simulink model "TBRe19_ECU_SequentialTests"  (R2017b)
settings: Solver=FixedStepDiscrete  StartTime=0.0  StopTime=inf  FixedStep=0.0001  RelTol=1e-3
PostLoadFcn:
  | model_init();
libraries: simulink x28
(part 2 of 22)

== system TBRe19_ECU_SequentialTests/DiagCAN3 ==
  note: ECU_Diag_ToCAN
  PostPL_Bus : Inport
  Bus Selector : BusSelector  OutputSignals=VFL_Data.DAL_Data.HAL_Data.HAL_Hardwired.Throttle1_Voltage,VFL_Data.DAL_Data.HAL_Data.HAL_Hardwired.Throttle2_Voltage,VFL_Data.DAL_Data.HAL_Data.HAL_Hardwired.Brake1_Pressure,VFL_Data.DAL_Data.HAL_Data.HAL_Hardwired.Brake2_Pressure
  Bus Selector1 : BusSelector  OutputSignals=VFL_Data.DAL_Data.Pedal_Box_Data.Brake1_Per,VFL_Data.DAL_Data.Pedal_Box_Data.Brake2_Per,VFL_Data.DAL_Data.Pedal_Box_Data.Brake_Percentage,VFL_Data.DAL_Data.Pedal_Box_Data.Throttle1_Per,VFL_Data.DAL_Data.Pedal_Box_Data.Throttle2_Per,VFL_Data.DAL_Data.Pedal_Box_Data.Throttle_Percentage
  Bus Selector2 : BusSelector  OutputSignals=VFL_Data.DAL_Data.HAL_Data.HAL_Hardwired.btnRTD_Input,VFL_Data.DAL_Data.HAL_Data.HAL_Hardwired.btnX_Input,VFL_Data.DAL_Data.HAL_Data.HAL_Hardwired.btnY_Input,VFL_Data.DAL_Data.HAL_Data.HAL_Hardwired.btnZ_Input,VFL_Data.DAL_Data.HAL_Data.HAL_Hardwired.Fan_Freq
  Bus Selector3 : BusSelector  OutputSignals=VFL_Data.DAL_Data.Pedal_Box_Data.Throttle_Bool,VFL_Data.DAL_Data.Pedal_Box_Data.Brake_Bool
  Bus Selector4 : BusSelector  OutputSignals=VFL_Data.DAL_Data.HAL_Data.HAL_Hardwired.AIRLow,VFL_Data.DAL_Data.HAL_Data.HAL_Hardwired.AIRHigh,VFL_Data.DAL_Data.Pedal_Box_Data.BPPS_Implausibility,VFL_Data.DAL_Data.Pedal_Box_Data.Pedal_Sensor_Fail,VFL_Data.DAL_Data.Pedal_Box_Data.APPS_Implausibility,VFL_Data.DAL_Data.Pedal_Box_Data.APPS_BP_Implausibility
  CanTx2 : S-Function  FunctionName=NsiCan_Tx_Ext  Parameters=data_can,channel,msg_name,ident,ident_type,dlc,signals,is_physical,is_canfd,is_crc  SFunctionDeploymentMode=off  EnableBusSupport=off  mask(MUXlink Can Tx){data_can=1;HIGH_SPEED;500Kbps;No;C:\Users\TBRe-admin\Documents\Database\TBRe19_DBC_190620.dbc;0;;;0;HIGH_SPEED;500Kbps;120 Ohm;C:\Users\TBRe-admin\Documents\Database\TBRe19_DBC_190517.dbc;0;;;0;HIGH_SPEED;1000Kbps;120 Ohm;D:\TOOLS\MUXLINK\R2011b\MUXlink\misc\BASE_CAN_MUXLAB4.dbc;0;;;0;HIGH_SPEED;500Kbps;120 Ohm;D:\TOOLS\MUXLINK\R2011b\MUXlink\misc\j1939_adapt.dbc;0;;;0;HIGH_SPEED;1000Kbps;No;D:\TOOLS\MUXLINK\R2011b\MUXlink\misc\BASE_CAN_MUXLAB4.dbc;0;;, channel=1, msg_name=VCU_Diagnostics, ident=0x700, ident_type=STD, dlc=4, signals=Shutdown_ECU;1;22;-1;1.000000;0.000000;_;Low_AIR_Status;1;20;-1;1.000000;0.000000;_;High_AIR_Status;1;21;1;1.000000;0.000000;_;BPPS_Implausibility;1;16;-1;1.000000;0.000000;_;Pedal_Sensor_Fail;1;24;8;1.000000;0.000000;_;APPS_Implausibility;1;17;1;1.000000;0.000000;_;APPS_BP_Implausibility;1;18;1;1.000000;0.000000;_;Shutdown_CarShutdown;1;23;1;1.000000;0.000000;_;LV_Battery_Warning;1;19;1;1.000000;0.000000;_;GearingRatio;1;8;8;0.100000;0.000000;_;Wheel_Size;1;0;8;0.100000;0.000000;m;Boost_on;1;34;-1;1.000000;0.000000;_;TC_on;1;33;-1;1.000000;0.000000;_;RegenBool;1;32;-1;1.000000;0.000000;_, is_physical=0, is_canfd=0, is_crc=0}
      mask prompts: data_can "data can"; msg_name "msg name"
      mask help: Transmit a frame on a CAN Channel.
      mask init:
      | NsiCan_Tx_Ext_InitializationFcn();
      settings: OpenFcn=NsiCan_Tx_Ext_OpenFcn();
      mask Help:
      | eval('block=get_param(gcb, ''RTWdata'');')
      | web([docroot '\toolbox\MUXlink\html\blocks/' block.MUXlink_BlockType '.html'])
      mask Callback data_can: NsiCan_Tx_Ext_ApplyFcn(1);
      mask Callback channel: NsiCan_Tx_Ext_ApplyFcn(2);
      mask Callback msg_name: NsiCan_Tx_Ext_ApplyFcn(3);
      mask Callback ident: NsiCan_Tx_Ext_ApplyFcn(4);
      mask Callback ident_type: NsiCan_Tx_Ext_ApplyFcn(5);
      mask Callback dlc: NsiCan_Tx_Ext_ApplyFcn(6);
      mask Callback signals: NsiCan_Tx_Ext_ApplyFcn(7);
      mask Callback is_physical: NsiCan_Tx_Ext_ApplyFcn(7);
      mask Callback is_canfd: NsiCan_Tx_Ext_ApplyFcn(7);
      mask Callback is_crc: NsiCan_Tx_Ext_ApplyFcn(7);
      mask Display: image(imread('nsi.bmp'));text(0.5, 0.3, 'TX_VCU_Diagnostics_CAN1', 'horizontalAlignment', 'center', 'verticalAlignment', 'base');plot([0.05 0.05 0.05 0.05 0.05 0.05 0.05 0.05 0.05 0.05]); port_label('input',1, 'Shutdown_ECU'); port_label('input',2, 'Low_AIR_Status'); port_label('input',3, 'High_AIR_Status'); port_label('input',4, 'BPPS_Implausibility'); port_label('input',5, 'Pedal_Sensor_Fail'); port_label('input',6, 'APPS_Implausibility'); port_label('input',7, 'APPS_BP_Implausibility'); port_label('input',8, 'Shutdown_CarShutdown'); port_label('input',9, 'LV_Battery_Warning'); port_label('input',10, 'GearingRatio'); port_label('input',11, 'Wheel_Size'); port_label('input',12, 'Boost_on'); port_label('input',13, 'TC_on'); port_label('input',14, 'RegenBool');
  CanTx6 : S-Function  FunctionName=NsiCan_Tx_Ext  Parameters=data_can,channel,msg_name,ident,ident_type,dlc,signals,is_physical,is_canfd,is_crc  SFunctionDeploymentMode=off  EnableBusSupport=off  mask(MUXlink Can Tx){data_can=1;HIGH_SPEED;500Kbps;No;C:\Users\TBRe-admin\Documents\Database\TBRe19_DBC_190621.dbc;0;;;0;HIGH_SPEED;500Kbps;120 Ohm;C:\Users\TBRe-admin\Documents\Database\TBRe19_DBC_190517.dbc;0;;;0;HIGH_SPEED;1000Kbps;120 Ohm;D:\TOOLS\MUXLINK\R2011b\MUXlink\misc\BASE_CAN_MUXLAB4.dbc;0;;;0;HIGH_SPEED;500Kbps;120 Ohm;D:\TOOLS\MUXLINK\R2011b\MUXlink\misc\j1939_adapt.dbc;0;;;0;HIGH_SPEED;1000Kbps;No;D:\TOOLS\MUXLINK\R2011b\MUXlink\misc\BASE_CAN_MUXLAB4.dbc;0;;, channel=1, msg_name=VCU_Pedal_Percentages, ident=0x702, ident_type=STD, dlc=7, signals=Brake1_Percentage;1;24;8;1.000000;0.000000;%;Brake2_Percentage;1;32;8;1.000000;0.000000;%;Brake_Percentage;1;48;8;1.000000;0.000000;%;BrakePot_Percentage;1;40;8;1.000000;0.000000;%;Throttle1_Percent;1;0;8;1.000000;0.000000;%;Throttle2_Percentage;1;8;8;1.000000;0.000000;%;Throttle_Percentage;1;16;8;1.000000;0.000000;%, is_physical=0, is_canfd=0, is_crc=0}
      mask prompts: data_can "data can"; msg_name "msg name"
      mask help: Transmit a frame on a CAN Channel.
      mask init:
      | NsiCan_Tx_Ext_InitializationFcn();
      settings: OpenFcn=NsiCan_Tx_Ext_OpenFcn();
      mask Help:
      | eval('block=get_param(gcb, ''RTWdata'');')
      | web([docroot '\toolbox\MUXlink\html\blocks/' block.MUXlink_BlockType '.html'])
      mask Callback data_can: NsiCan_Tx_Ext_ApplyFcn(1);
      mask Callback channel: NsiCan_Tx_Ext_ApplyFcn(2);
      mask Callback msg_name: NsiCan_Tx_Ext_ApplyFcn(3);
      mask Callback ident: NsiCan_Tx_Ext_ApplyFcn(4);
      mask Callback ident_type: NsiCan_Tx_Ext_ApplyFcn(5);
      mask Callback dlc: NsiCan_Tx_Ext_ApplyFcn(6);
      mask Callback signals: NsiCan_Tx_Ext_ApplyFcn(7);
      mask Callback is_physical: NsiCan_Tx_Ext_ApplyFcn(7);
      mask Callback is_canfd: NsiCan_Tx_Ext_ApplyFcn(7);
      mask Callback is_crc: NsiCan_Tx_Ext_ApplyFcn(7);
      mask Display: image(imread('nsi.bmp'));text(0.5, 0.1, 'TX_VCU_Pedal_Percentages_CAN1', 'horizontalAlignment', 'center', 'verticalAlignment', 'base');plot([0.05 0.05 0.05 0.05 0.05 0.05 0.05 0.05 0.05 0.05]); port_label('input',1, 'Brake1_Percentage'); port_label('input',2, 'Brake2_Percentage'); port_label('input',3, 'Brake_Percentage'); port_label('input',4, 'BrakePot_Percentage'); port_label('input',5, 'Throttle1_Percent'); port_label('input',6, 'Throttle2_Percentage'); port_label('input',7, 'Throttle_Percentage');
  CanTx7 : S-Function  FunctionName=NsiCan_Tx_Ext  Parameters=data_can,channel,msg_name,ident,ident_type,dlc,signals,is_physical,is_canfd,is_crc  SFunctionDeploymentMode=off  EnableBusSupport=off  mask(MUXlink Can Tx){data_can=1;HIGH_SPEED;500Kbps;No;C:\Users\TBRe-admin\Documents\Database\TBRe19_DBC_190621.dbc;0;;;0;HIGH_SPEED;500Kbps;120 Ohm;C:\Users\TBRe-admin\Documents\Database\TBRe19_DBC_190517.dbc;0;;;0;HIGH_SPEED;1000Kbps;120 Ohm;D:\TOOLS\MUXLINK\R2011b\MUXlink\misc\BASE_CAN_MUXLAB4.dbc;0;;;0;HIGH_SPEED;500Kbps;120 Ohm;D:\TOOLS\MUXLINK\R2011b\MUXlink\misc\j1939_adapt.dbc;0;;;0;HIGH_SPEED;1000Kbps;No;D:\TOOLS\MUXLINK\R2011b\MUXlink\misc\BASE_CAN_MUXLAB4.dbc;0;;, channel=1, msg_name=VCU_HW_IO, ident=0x701, ident_type=STD, dlc=4, signals=Console_RTD;1;0;1;1.000000;0.000000;Bool;Console_X;1;3;1;1.000000;0.000000;Bool;Consle_Y;1;2;-1;1.000000;0.000000;Bool;Console_Z;1;1;-1;1.000000;0.000000;_;Coolant_Pump_Fan;1;5;1;1.000000;0.000000;_;Coolant_AccyFan;1;6;-1;1.000000;0.000000;_;Buzzer;1;7;1;1.000000;0.000000;_;LV_Battery_Voltage;1;16;16;1.000000;0.000000;mV;LV_Battery_SOC;1;8;8;1.000000;0.000000;_;AccyFanFreq;1;32;8;1.000000;0.000000;Hz, is_physical=0, is_canfd=0, is_crc=0}
      mask prompts: data_can "data can"; msg_name "msg name"
      mask help: Transmit a frame on a CAN Channel.
      mask init:
      | NsiCan_Tx_Ext_InitializationFcn();
      settings: OpenFcn=NsiCan_Tx_Ext_OpenFcn();
      mask Help:
      | eval('block=get_param(gcb, ''RTWdata'');')
      | web([docroot '\toolbox\MUXlink\html\blocks/' block.MUXlink_BlockType '.html'])
      mask Callback data_can: NsiCan_Tx_Ext_ApplyFcn(1);
      mask Callback channel: NsiCan_Tx_Ext_ApplyFcn(2);
      mask Callback msg_name: NsiCan_Tx_Ext_ApplyFcn(3);
      mask Callback ident: NsiCan_Tx_Ext_ApplyFcn(4);
      mask Callback ident_type: NsiCan_Tx_Ext_ApplyFcn(5);
      mask Callback dlc: NsiCan_Tx_Ext_ApplyFcn(6);
      mask Callback signals: NsiCan_Tx_Ext_ApplyFcn(7);
      mask Callback is_physical: NsiCan_Tx_Ext_ApplyFcn(7);
      mask Callback is_canfd: NsiCan_Tx_Ext_ApplyFcn(7);
      mask Callback is_crc: NsiCan_Tx_Ext_ApplyFcn(7);
      mask Display: image(imread('nsi.bmp'));text(0.5, 0.3, 'TX_VCU_HW_IO_CAN1', 'horizontalAlignment', 'center', 'verticalAlignment', 'base');plot([0.05 0.05 0.05 0.05 0.05 0.05 0.05 0.05 0.05 0.05]); port_label('input',1, 'Console_RTD'); port_label('input',2, 'Console_X'); port_label('input',3, 'Consle_Y'); port_label('input',4, 'Console_Z'); port_label('input',5, 'Coolant_Pump_Fan'); port_label('input',6, 'Coolant_AccyFan'); port_label('input',7, 'Buzzer'); port_label('input',8, 'LV_Battery_Voltage'); port_label('input',9, 'LV_Battery_SOC'); port_label('input',10, 'AccyFanFreq');
  CanTx8 : S-Function  FunctionName=NsiCan_Tx_Ext  Parameters=data_can,channel,msg_name,ident,ident_type,dlc,signals,is_physical,is_canfd,is_crc  SFunctionDeploymentMode=off  EnableBusSupport=off  mask(MUXlink Can Tx){data_can=1;HIGH_SPEED;500Kbps;No;C:\Users\TBRe-admin\Documents\Database\TBRe19_DBC_190620.dbc;0;;;0;HIGH_SPEED;500Kbps;120 Ohm;C:\Users\TBRe-admin\Documents\Database\TBRe19_DBC_190517.dbc;0;;;0;HIGH_SPEED;1000Kbps;120 Ohm;D:\TOOLS\MUXLINK\R2011b\MUXlink\misc\BASE_CAN_MUXLAB4.dbc;0;;;0;HIGH_SPEED;500Kbps;120 Ohm;D:\TOOLS\MUXLINK\R2011b\MUXlink\misc\j1939_adapt.dbc;0;;;0;HIGH_SPEED;1000Kbps;No;D:\TOOLS\MUXLINK\R2011b\MUXlink\misc\BASE_CAN_MUXLAB4.dbc;0;;, channel=1, msg_name=VCU_Vehicle_Functionality, ident=0x704, ident_type=STD, dlc=4, signals=Tractive_System_Startup;1;24;1;1.000000;0.000000;_;Throttle_Bool;1;25;1;1.000000;0.000000;_;MCU_NMT_Mode;1;16;8;1.000000;0.000000;_;Control_Word;1;0;8;1.000000;0.000000;_;Vehicle_Operation;1;8;8;1.000000;0.000000;_;Brake_Bool;1;26;1;1.000000;0.000000;_, is_physical=0, is_canfd=0, is_crc=0}
      mask prompts: data_can "data can"; msg_name "msg name"
      mask help: Transmit a frame on a CAN Channel.
      mask init:
      | NsiCan_Tx_Ext_InitializationFcn();
      settings: OpenFcn=NsiCan_Tx_Ext_OpenFcn();
      mask Help:
      | eval('block=get_param(gcb, ''RTWdata'');')
      | web([docroot '\toolbox\MUXlink\html\blocks/' block.MUXlink_BlockType '.html'])
      mask Callback data_can: NsiCan_Tx_Ext_ApplyFcn(1);
      mask Callback channel: NsiCan_Tx_Ext_ApplyFcn(2);
      mask Callback msg_name: NsiCan_Tx_Ext_ApplyFcn(3);
      mask Callback ident: NsiCan_Tx_Ext_ApplyFcn(4);
      mask Callback ident_type: NsiCan_Tx_Ext_ApplyFcn(5);
      mask Callback dlc: NsiCan_Tx_Ext_ApplyFcn(6);
      mask Callback signals: NsiCan_Tx_Ext_ApplyFcn(7);
      mask Callback is_physical: NsiCan_Tx_Ext_ApplyFcn(7);
      mask Callback is_canfd: NsiCan_Tx_Ext_ApplyFcn(7);
      mask Callback is_crc: NsiCan_Tx_Ext_ApplyFcn(7);
      mask Display: image(imread('nsi.bmp'));text(0.5, 0.3, 'TX_VCU_Vehicle_Functionality_CAN1', 'horizontalAlignment', 'center', 'verticalAlignment', 'base');plot([0.05 0.05 0.05 0.05 0.05 0.05 0.05 0.05 0.05 0.05]); port_label('input',1, 'Tractive_System_Startup'); port_label('input',2, 'Throttle_Bool'); port_label('input',3, 'MCU_NMT_Mode'); port_label('input',4, 'Control_Word'); port_label('input',5, 'Vehicle_Operation'); port_label('input',6, 'Brake_Bool');
  CanTx9 : S-Function  FunctionName=NsiCan_Tx_Ext  Parameters=data_can,channel,msg_name,ident,ident_type,dlc,signals,is_physical,is_canfd,is_crc  SFunctionDeploymentMode=off  EnableBusSupport=off  mask(MUXlink Can Tx){data_can=1;HIGH_SPEED;500Kbps;No;C:\Users\TBRe-admin\Documents\Database\TBRe19_DBC_190621.dbc;0;;;0;HIGH_SPEED;500Kbps;120 Ohm;C:\Users\TBRe-admin\Documents\Database\TBRe19_DBC_190517.dbc;0;;;0;HIGH_SPEED;1000Kbps;120 Ohm;D:\TOOLS\MUXLINK\R2011b\MUXlink\misc\BASE_CAN_MUXLAB4.dbc;0;;;0;HIGH_SPEED;500Kbps;120 Ohm;D:\TOOLS\MUXLINK\R2011b\MUXlink\misc\j1939_adapt.dbc;0;;;0;HIGH_SPEED;1000Kbps;No;D:\TOOLS\MUXLINK\R2011b\MUXlink\misc\BASE_CAN_MUXLAB4.dbc;0;;, channel=1, msg_name=VCU_Pedal_Voltages, ident=0x703, ident_type=STD, dlc=8, signals=Throttle1_Voltage;1;0;16;1.000000;0.000000;mV;Throttle2_Voltage;1;32;16;1.000000;0.000000;mV;Brake1_Voltage;1;16;16;1.000000;0.000000;mV;Brake2_Voltage;1;48;16;1.000000;0.000000;mV, is_physical=0, is_canfd=0, is_crc=0}
      mask prompts: data_can "data can"; msg_name "msg name"
      mask help: Transmit a frame on a CAN Channel.
      mask init:
      | NsiCan_Tx_Ext_InitializationFcn();
      settings: OpenFcn=NsiCan_Tx_Ext_OpenFcn();
      mask Help:
      | eval('block=get_param(gcb, ''RTWdata'');')
      | web([docroot '\toolbox\MUXlink\html\blocks/' block.MUXlink_BlockType '.html'])
      mask Callback data_can: NsiCan_Tx_Ext_ApplyFcn(1);
      mask Callback channel: NsiCan_Tx_Ext_ApplyFcn(2);
      mask Callback msg_name: NsiCan_Tx_Ext_ApplyFcn(3);
      mask Callback ident: NsiCan_Tx_Ext_ApplyFcn(4);
      mask Callback ident_type: NsiCan_Tx_Ext_ApplyFcn(5);
      mask Callback dlc: NsiCan_Tx_Ext_ApplyFcn(6);
      mask Callback signals: NsiCan_Tx_Ext_ApplyFcn(7);
      mask Callback is_physical: NsiCan_Tx_Ext_ApplyFcn(7);
      mask Callback is_canfd: NsiCan_Tx_Ext_ApplyFcn(7);
      mask Callback is_crc: NsiCan_Tx_Ext_ApplyFcn(7);
      mask Display: image(imread('nsi.bmp'));text(0.5, 0.3, 'TX_VCU_Pedal_Voltages_CAN1', 'horizontalAlignment', 'center', 'verticalAlignment', 'base');plot([0.05 0.05 0.05 0.05 0.05 0.05 0.05 0.05 0.05 0.05]); port_label('input',1, 'Throttle1_Voltage'); port_label('input',2, 'Throttle2_Voltage'); port_label('input',3, 'Brake1_Voltage'); port_label('input',4, 'Brake2_Voltage');
  Data Type Conversion{2..11,14,17,21..22,26..30} (19 alike) : DataTypeConversion
  Init : Subsystem  mask(System Initialize){}
      mask help: Add code to a systems Initialize function
      settings: CopyFcn=cccopyfcn(gcb)  OpenFcn=ccopenfcn('System Initialize Function')
      mask Help: This block contains text fields to insert custom user code sections at the declaration, execution and exit sections of the systems initialize function.  By placing this block inside a subsytem, the custom user code will appear in that subsystems function.
      mask Display: disp('I()')
  Task : S-Function  FunctionName=NsiSys_TaskREF  Parameters=task_initialised,task_periodic, task_sampletime,task_name,task_event,task_offset  SFunctionDeploymentMode=off  EnableBusSupport=off  mask(task definition){task_initialised=on, task_periodic=on, task_sampletime=[0.1], task_offset=0.01, task_name=DiagCAN3, task_event=on}
      mask prompts: task_initialised "task initialised"; task_periodic "Is Periodic"; task_sampletime "Task sample time"; task_offset "Task Offset"; task_name "Task name"; task_event "Is event"
      mask help:
      | Permit to provide all parameters associated to a MUXLINK task.
      | Task can be executed periodicaly and/or on event detection.
      | If task is periodic:
      | Task sample time specify the execution period in mS [0.001   6000]
      | Task Offset specify the offset applied to the execution period
      | Task Offset < Task sample time
      mask init:
      | NsiSys_TaskREF_InitializationFcn();
      settings: OpenFcn=NsiSys_Task_OpenFcn();
      mask Callback task_initialised: NsiSys_TaskREF_ApplyFcn(1);
      mask Callback task_periodic: NsiSys_TaskREF_ApplyFcn(2);
      mask Callback task_sampletime: NsiSys_TaskREF_ApplyFcn(3);
      mask Callback task_offset: NsiSys_TaskREF_ApplyFcn(6);
      mask Callback task_name: NsiSys_TaskREF_ApplyFcn(4);
      mask Callback task_event: NsiSys_TaskREF_ApplyFcn(5);
      mask Display: text(0.5, 0.8, 't()', 'horizontalAlignment', 'center', 'verticalAlignment', 'base');text(0.5, 0.2, '/ 100.0ms / 10.0ms /', 'horizontalAlignment', 'center', 'verticalAlignment', 'base');text(0.5, 0.4, 'Event', 'horizontalAlignment', 'center', 'verticalAlignment', 'base');
  UsbRx : S-Function  FunctionName=NsiUsb_Rx  Parameters=signame,sigtype,resolution,offset,unite,value,is_trigger  SFunctionDeploymentMode=off  EnableBusSupport=off  mask(MUXlink Usb Rx){signame=Wheel_Size, sigtype=Unsigned Byte, resolution=1, offset=0, unite=mm, value=450, is_trigger=off}
      mask prompts: signame "Signal name :"; sigtype "Signal type :"; resolution "Resolution :"; offset "Offset :"; unite "Unit :"; value "Default value :"; is_trigger "Is trigger ?"
      mask help: Receive a frame on the USB Channel.
      mask init:
      | NsiUsb_Rx_InitializationFcn();
      settings: OpenFcn=NsiUsb_Rx_OpenFcn();
      mask Help:
      | eval('block=get_param(gcb, ''RTWdata'');')
      | web([docroot '\toolbox\MUXlink\html\blocks/' block.MUXlink_BlockType '.html'])
      mask Callback signame: NsiUsb_Rx_ApplyFcn(1);
      mask TypeOptions sigtype: Boolean | Signed Byte | Unsigned Byte | Signed Word | Unsigned Word | Signed Double Word | Unsigned Double Word | Single Float | Double Float
      mask Callback sigtype: NsiUsb_Rx_ApplyFcn(2);
      mask Callback resolution: NsiUsb_Rx_ApplyFcn(3);
      mask Callback offset: NsiUsb_Rx_ApplyFcn(4);
      mask Callback unite: NsiUsb_Rx_ApplyFcn(5);
      mask Callback value: NsiUsb_Rx_ApplyFcn(6);
      mask Callback is_trigger: NsiUsb_Rx_ApplyFcn(7);
      mask Display: image(imread('nsi.bmp'));text(0.5, 0.2, 'USB Rx', 'horizontalAlignment', 'center', 'verticalAlignment', 'base');plot([0.05 0.05 0.05 0.05 0.05 0.05 0.05 0.05 0.05 0.05]);port_label('output',1, 'Wheel_Size');
  UsbRx1 : S-Function  FunctionName=NsiUsb_Rx  Parameters=signame,sigtype,resolution,offset,unite,value,is_trigger  SFunctionDeploymentMode=off  EnableBusSupport=off  mask(MUXlink Usb Rx){signame=Gearing_Ratio, sigtype=Unsigned Byte, resolution=1, offset=0, unite=ratio, value=3, is_trigger=off}
      mask prompts: signame "Signal name :"; sigtype "Signal type :"; resolution "Resolution :"; offset "Offset :"; unite "Unit :"; value "Default value :"; is_trigger "Is trigger ?"
      mask help: Receive a frame on the USB Channel.
      mask init:
      | NsiUsb_Rx_InitializationFcn();
      settings: OpenFcn=NsiUsb_Rx_OpenFcn();
      mask Help:
      | eval('block=get_param(gcb, ''RTWdata'');')
      | web([docroot '\toolbox\MUXlink\html\blocks/' block.MUXlink_BlockType '.html'])
      mask Callback signame: NsiUsb_Rx_ApplyFcn(1);
      mask TypeOptions sigtype: Boolean | Signed Byte | Unsigned Byte | Signed Word | Unsigned Word | Signed Double Word | Unsigned Double Word | Single Float | Double Float
      mask Callback sigtype: NsiUsb_Rx_ApplyFcn(2);
      mask Callback resolution: NsiUsb_Rx_ApplyFcn(3);
      mask Callback offset: NsiUsb_Rx_ApplyFcn(4);
      mask Callback unite: NsiUsb_Rx_ApplyFcn(5);
      mask Callback value: NsiUsb_Rx_ApplyFcn(6);
      mask Callback is_trigger: NsiUsb_Rx_ApplyFcn(7);
      mask Display: image(imread('nsi.bmp'));text(0.5, 0.2, 'USB Rx', 'horizontalAlignment', 'center', 'verticalAlignment', 'base');plot([0.05 0.05 0.05 0.05 0.05 0.05 0.05 0.05 0.05 0.05]);port_label('output',1, 'Gearing_Ratio');
  wires:
  Data Type Conversion17/1 -> CanTx8/2
  Data Type Conversion14/1 -> CanTx6/1
  Data Type Conversion22/1 -> CanTx7/10
  Data Type Conversion28/1 -> CanTx2/4
  Data Type Conversion26/1 -> CanTx2/3
  Data Type Conversion6/1 -> CanTx9/4
  Data Type Conversion11/1 -> CanTx2/5
  Data Type Conversion3/1 -> CanTx9/3
  Data Type Conversion4/1 -> CanTx9/1
  Bus Selector1/6 -> Data Type Conversion5/1  "<Throttle_Percentage>"
  Data Type Conversion21/1 -> CanTx8/6
  Bus Selector/4 -> Data Type Conversion6/1  "<Brake2_Pressure>"
  UsbRx1/1 -> CanTx2/10
  Bus Selector2/4 -> CanTx7/4  "<btnZ_Input>"
  Bus Selector4/3 -> Data Type Conversion28/1  "<BPPS_Implausibility>"
  Bus Selector4/1 -> Data Type Conversion27/1  "<AIRLow>"
  Data Type Conversion9/1 -> CanTx6/6
  Bus Selector1/1 -> Data Type Conversion14/1  "<Brake1_Per>"
  UsbRx/1 -> CanTx2/11
  Bus Selector4/2 -> Data Type Conversion26/1  "<AIRHigh>"
  Data Type Conversion27/1 -> CanTx2/2
  Data Type Conversion29/1 -> CanTx2/6
  Data Type Conversion5/1 -> CanTx6/7
  Data Type Conversion7/1 -> CanTx6/2
  Data Type Conversion8/1 -> CanTx6/3
  Bus Selector1/3 -> Data Type Conversion8/1  "<Brake_Percentage>"
  Bus Selector4/6 -> Data Type Conversion30/1  "<APPS_BP_Implausibility>"
  Bus Selector/1 -> Data Type Conversion4/1  "<Throttle1_Voltage>"
  Bus Selector4/5 -> Data Type Conversion29/1  "<APPS_Implausibility>"
  Bus Selector/2 -> Data Type Conversion2/1  "<Throttle2_Voltage>"
  Bus Selector2/1 -> CanTx7/1  "<btnRTD_Input>"
  PostPL_Bus/1 -> Bus Selector/1, Bus Selector1/1, Bus Selector2/1, Bus Selector4/1, Bus Selector3/1
  Bus Selector1/5 -> Data Type Conversion9/1  "<Throttle2_Per>"
  Bus Selector1/2 -> Data Type Conversion7/1  "<Brake2_Per>"
  Data Type Conversion10/1 -> CanTx6/5
  Bus Selector1/4 -> Data Type Conversion10/1  "<Throttle1_Per>"
  Data Type Conversion30/1 -> CanTx2/7
  Bus Selector2/5 -> Data Type Conversion22/1  "<Fan_Freq>"
  Bus Selector3/1 -> Data Type Conversion17/1  "<Throttle_Bool>"
  Bus Selector3/2 -> Data Type Conversion21/1  "<Brake_Bool>"
  Data Type Conversion2/1 -> CanTx9/2
  Bus Selector/3 -> Data Type Conversion3/1  "<Brake1_Pressure>"
  Bus Selector2/2 -> CanTx7/2  "<btnX_Input>"
  Bus Selector4/4 -> Data Type Conversion11/1  "<Pedal_Sensor_Fail>"
  Bus Selector2/3 -> CanTx7/3  "<btnY_Input>"

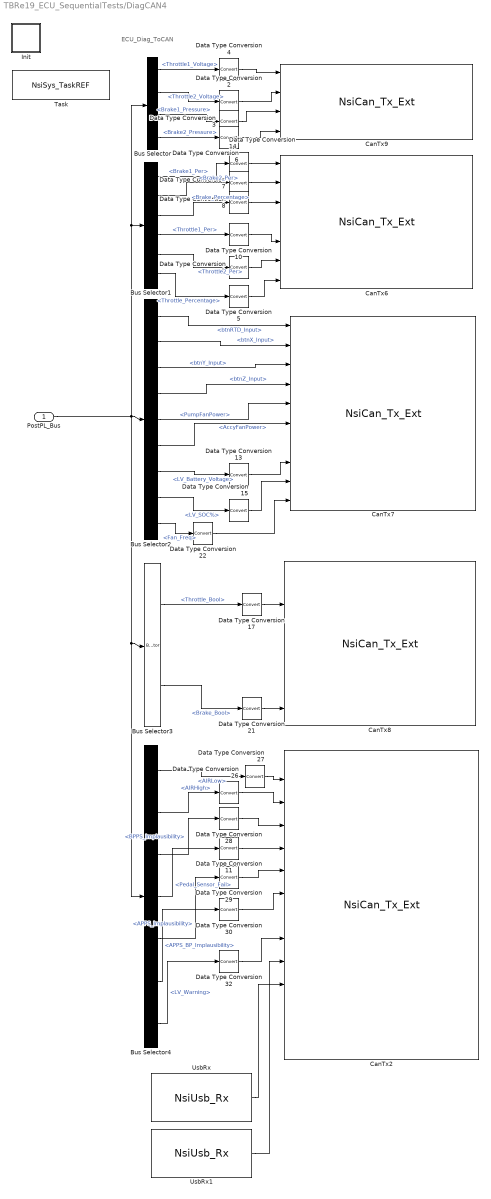
== system TBRe19_ECU_SequentialTests/DiagCAN4 ==
  note: ECU_Diag_ToCAN
  PostPL_Bus : Inport
  Bus Selector : BusSelector  OutputSignals=VFL_Data.DAL_Data.HAL_Data.HAL_Hardwired.Throttle1_Voltage,VFL_Data.DAL_Data.HAL_Data.HAL_Hardwired.Throttle2_Voltage,VFL_Data.DAL_Data.HAL_Data.HAL_Hardwired.Brake1_Pressure,VFL_Data.DAL_Data.HAL_Data.HAL_Hardwired.Brake2_Pressure
  Bus Selector1 : BusSelector  OutputSignals=VFL_Data.DAL_Data.Pedal_Box_Data.Brake1_Per,VFL_Data.DAL_Data.Pedal_Box_Data.Brake2_Per,VFL_Data.DAL_Data.Pedal_Box_Data.Brake_Percentage,VFL_Data.DAL_Data.Pedal_Box_Data.Throttle1_Per,VFL_Data.DAL_Data.Pedal_Box_Data.Throttle2_Per,VFL_Data.DAL_Data.Pedal_Box_Data.Throttle_Percentage
  Bus Selector2 : BusSelector  OutputSignals=VFL_Data.DAL_Data.HAL_Data.HAL_Hardwired.btnRTD_Input,VFL_Data.DAL_Data.HAL_Data.HAL_Hardwired.btnX_Input,VFL_Data.DAL_Data.HAL_Data.HAL_Hardwired.btnY_Input,VFL_Data.DAL_Data.HAL_Data.HAL_Hardwired.btnZ_Input,Hardwired_Peripherals.PumpFanPower,Hardwired_Peripherals.AccyFanPower,VFL_Data.DAL_Data.LV_Battery.LV_Battery_Voltage,VFL_Data.DAL_Data.LV_Battery.LV_SOC%,VFL_Data.DAL_Data.HAL_Data.HAL_Hardwired.Fan_Freq
  Bus Selector3 : BusSelector  OutputSignals=VFL_Data.DAL_Data.Pedal_Box_Data.Throttle_Bool,VFL_Data.DAL_Data.Pedal_Box_Data.Brake_Bool
  Bus Selector4 : BusSelector  OutputSignals=VFL_Data.DAL_Data.HAL_Data.HAL_Hardwired.AIRLow,VFL_Data.DAL_Data.HAL_Data.HAL_Hardwired.AIRHigh,VFL_Data.DAL_Data.Pedal_Box_Data.BPPS_Implausibility,VFL_Data.DAL_Data.Pedal_Box_Data.Pedal_Sensor_Fail,VFL_Data.DAL_Data.Pedal_Box_Data.APPS_Implausibility,VFL_Data.DAL_Data.Pedal_Box_Data.APPS_BP_Implausibility,VFL_Data.DAL_Data.LV_Battery.LV_Warning
  CanTx2 : S-Function  FunctionName=NsiCan_Tx_Ext  Parameters=data_can,channel,msg_name,ident,ident_type,dlc,signals,is_physical,is_canfd,is_crc  SFunctionDeploymentMode=off  EnableBusSupport=off  mask(MUXlink Can Tx){data_can=1;HIGH_SPEED;500Kbps;No;C:\Users\TBRe-admin\Documents\Database\TBRe19_DBC_190620.dbc;0;;;0;HIGH_SPEED;500Kbps;120 Ohm;C:\Users\TBRe-admin\Documents\Database\TBRe19_DBC_190517.dbc;0;;;0;HIGH_SPEED;1000Kbps;120 Ohm;D:\TOOLS\MUXLINK\R2011b\MUXlink\misc\BASE_CAN_MUXLAB4.dbc;0;;;0;HIGH_SPEED;500Kbps;120 Ohm;D:\TOOLS\MUXLINK\R2011b\MUXlink\misc\j1939_adapt.dbc;0;;;0;HIGH_SPEED;1000Kbps;No;D:\TOOLS\MUXLINK\R2011b\MUXlink\misc\BASE_CAN_MUXLAB4.dbc;0;;, channel=1, msg_name=VCU_Diagnostics, ident=0x700, ident_type=STD, dlc=4, signals=Shutdown_ECU;1;22;-1;1.000000;0.000000;_;Low_AIR_Status;1;20;-1;1.000000;0.000000;_;High_AIR_Status;1;21;1;1.000000;0.000000;_;BPPS_Implausibility;1;16;-1;1.000000;0.000000;_;Pedal_Sensor_Fail;1;24;8;1.000000;0.000000;_;APPS_Implausibility;1;17;1;1.000000;0.000000;_;APPS_BP_Implausibility;1;18;1;1.000000;0.000000;_;Shutdown_CarShutdown;1;23;1;1.000000;0.000000;_;LV_Battery_Warning;1;19;1;1.000000;0.000000;_;GearingRatio;1;8;8;0.100000;0.000000;_;Wheel_Size;1;0;8;0.100000;0.000000;m;Boost_on;1;34;-1;1.000000;0.000000;_;TC_on;1;33;-1;1.000000;0.000000;_;RegenBool;1;32;-1;1.000000;0.000000;_, is_physical=0, is_canfd=0, is_crc=0}
      mask prompts: data_can "data can"; msg_name "msg name"
      mask help: Transmit a frame on a CAN Channel.
      mask init:
      | NsiCan_Tx_Ext_InitializationFcn();
      settings: OpenFcn=NsiCan_Tx_Ext_OpenFcn();
      mask Help:
      | eval('block=get_param(gcb, ''RTWdata'');')
      | web([docroot '\toolbox\MUXlink\html\blocks/' block.MUXlink_BlockType '.html'])
      mask Callback data_can: NsiCan_Tx_Ext_ApplyFcn(1);
      mask Callback channel: NsiCan_Tx_Ext_ApplyFcn(2);
      mask Callback msg_name: NsiCan_Tx_Ext_ApplyFcn(3);
      mask Callback ident: NsiCan_Tx_Ext_ApplyFcn(4);
      mask Callback ident_type: NsiCan_Tx_Ext_ApplyFcn(5);
      mask Callback dlc: NsiCan_Tx_Ext_ApplyFcn(6);
      mask Callback signals: NsiCan_Tx_Ext_ApplyFcn(7);
      mask Callback is_physical: NsiCan_Tx_Ext_ApplyFcn(7);
      mask Callback is_canfd: NsiCan_Tx_Ext_ApplyFcn(7);
      mask Callback is_crc: NsiCan_Tx_Ext_ApplyFcn(7);
      mask Display: image(imread('nsi.bmp'));text(0.5, 0.3, 'TX_VCU_Diagnostics_CAN1', 'horizontalAlignment', 'center', 'verticalAlignment', 'base');plot([0.05 0.05 0.05 0.05 0.05 0.05 0.05 0.05 0.05 0.05]); port_label('input',1, 'Shutdown_ECU'); port_label('input',2, 'Low_AIR_Status'); port_label('input',3, 'High_AIR_Status'); port_label('input',4, 'BPPS_Implausibility'); port_label('input',5, 'Pedal_Sensor_Fail'); port_label('input',6, 'APPS_Implausibility'); port_label('input',7, 'APPS_BP_Implausibility'); port_label('input',8, 'Shutdown_CarShutdown'); port_label('input',9, 'LV_Battery_Warning'); port_label('input',10, 'GearingRatio'); port_label('input',11, 'Wheel_Size'); port_label('input',12, 'Boost_on'); port_label('input',13, 'TC_on'); port_label('input',14, 'RegenBool');
  CanTx6 : S-Function  FunctionName=NsiCan_Tx_Ext  Parameters=data_can,channel,msg_name,ident,ident_type,dlc,signals,is_physical,is_canfd,is_crc  SFunctionDeploymentMode=off  EnableBusSupport=off  mask(MUXlink Can Tx){data_can=1;HIGH_SPEED;500Kbps;No;C:\Users\TBRe-admin\Documents\Database\TBRe19_DBC_190621.dbc;0;;;0;HIGH_SPEED;500Kbps;120 Ohm;C:\Users\TBRe-admin\Documents\Database\TBRe19_DBC_190517.dbc;0;;;0;HIGH_SPEED;1000Kbps;120 Ohm;D:\TOOLS\MUXLINK\R2011b\MUXlink\misc\BASE_CAN_MUXLAB4.dbc;0;;;0;HIGH_SPEED;500Kbps;120 Ohm;D:\TOOLS\MUXLINK\R2011b\MUXlink\misc\j1939_adapt.dbc;0;;;0;HIGH_SPEED;1000Kbps;No;D:\TOOLS\MUXLINK\R2011b\MUXlink\misc\BASE_CAN_MUXLAB4.dbc;0;;, channel=1, msg_name=VCU_Pedal_Percentages, ident=0x702, ident_type=STD, dlc=7, signals=Brake1_Percentage;1;24;8;1.000000;0.000000;%;Brake2_Percentage;1;32;8;1.000000;0.000000;%;Brake_Percentage;1;48;8;1.000000;0.000000;%;BrakePot_Percentage;1;40;8;1.000000;0.000000;%;Throttle1_Percent;1;0;8;1.000000;0.000000;%;Throttle2_Percentage;1;8;8;1.000000;0.000000;%;Throttle_Percentage;1;16;8;1.000000;0.000000;%, is_physical=0, is_canfd=0, is_crc=0}
      mask prompts: data_can "data can"; msg_name "msg name"
      mask help: Transmit a frame on a CAN Channel.
      mask init:
      | NsiCan_Tx_Ext_InitializationFcn();
      settings: OpenFcn=NsiCan_Tx_Ext_OpenFcn();
      mask Help:
      | eval('block=get_param(gcb, ''RTWdata'');')
      | web([docroot '\toolbox\MUXlink\html\blocks/' block.MUXlink_BlockType '.html'])
      mask Callback data_can: NsiCan_Tx_Ext_ApplyFcn(1);
      mask Callback channel: NsiCan_Tx_Ext_ApplyFcn(2);
      mask Callback msg_name: NsiCan_Tx_Ext_ApplyFcn(3);
      mask Callback ident: NsiCan_Tx_Ext_ApplyFcn(4);
      mask Callback ident_type: NsiCan_Tx_Ext_ApplyFcn(5);
      mask Callback dlc: NsiCan_Tx_Ext_ApplyFcn(6);
      mask Callback signals: NsiCan_Tx_Ext_ApplyFcn(7);
      mask Callback is_physical: NsiCan_Tx_Ext_ApplyFcn(7);
      mask Callback is_canfd: NsiCan_Tx_Ext_ApplyFcn(7);
      mask Callback is_crc: NsiCan_Tx_Ext_ApplyFcn(7);
      mask Display: image(imread('nsi.bmp'));text(0.5, 0.1, 'TX_VCU_Pedal_Percentages_CAN1', 'horizontalAlignment', 'center', 'verticalAlignment', 'base');plot([0.05 0.05 0.05 0.05 0.05 0.05 0.05 0.05 0.05 0.05]); port_label('input',1, 'Brake1_Percentage'); port_label('input',2, 'Brake2_Percentage'); port_label('input',3, 'Brake_Percentage'); port_label('input',4, 'BrakePot_Percentage'); port_label('input',5, 'Throttle1_Percent'); port_label('input',6, 'Throttle2_Percentage'); port_label('input',7, 'Throttle_Percentage');
  CanTx7 : S-Function  FunctionName=NsiCan_Tx_Ext  Parameters=data_can,channel,msg_name,ident,ident_type,dlc,signals,is_physical,is_canfd,is_crc  SFunctionDeploymentMode=off  EnableBusSupport=off  mask(MUXlink Can Tx){data_can=1;HIGH_SPEED;500Kbps;No;C:\Users\TBRe-admin\Documents\Database\TBRe19_DBC_190621.dbc;0;;;0;HIGH_SPEED;500Kbps;120 Ohm;C:\Users\TBRe-admin\Documents\Database\TBRe19_DBC_190517.dbc;0;;;0;HIGH_SPEED;1000Kbps;120 Ohm;D:\TOOLS\MUXLINK\R2011b\MUXlink\misc\BASE_CAN_MUXLAB4.dbc;0;;;0;HIGH_SPEED;500Kbps;120 Ohm;D:\TOOLS\MUXLINK\R2011b\MUXlink\misc\j1939_adapt.dbc;0;;;0;HIGH_SPEED;1000Kbps;No;D:\TOOLS\MUXLINK\R2011b\MUXlink\misc\BASE_CAN_MUXLAB4.dbc;0;;, channel=1, msg_name=VCU_HW_IO, ident=0x701, ident_type=STD, dlc=4, signals=Console_RTD;1;0;1;1.000000;0.000000;Bool;Console_X;1;3;1;1.000000;0.000000;Bool;Consle_Y;1;2;-1;1.000000;0.000000;Bool;Console_Z;1;1;-1;1.000000;0.000000;_;Coolant_Pump_Fan;1;5;1;1.000000;0.000000;_;Coolant_AccyFan;1;6;-1;1.000000;0.000000;_;Buzzer;1;7;1;1.000000;0.000000;_;LV_Battery_Voltage;1;16;16;1.000000;0.000000;mV;LV_Battery_SOC;1;8;8;1.000000;0.000000;_;AccyFanFreq;1;32;8;1.000000;0.000000;Hz, is_physical=0, is_canfd=0, is_crc=0}
      mask prompts: data_can "data can"; msg_name "msg name"
      mask help: Transmit a frame on a CAN Channel.
      mask init:
      | NsiCan_Tx_Ext_InitializationFcn();
      settings: OpenFcn=NsiCan_Tx_Ext_OpenFcn();
      mask Help:
      | eval('block=get_param(gcb, ''RTWdata'');')
      | web([docroot '\toolbox\MUXlink\html\blocks/' block.MUXlink_BlockType '.html'])
      mask Callback data_can: NsiCan_Tx_Ext_ApplyFcn(1);
      mask Callback channel: NsiCan_Tx_Ext_ApplyFcn(2);
      mask Callback msg_name: NsiCan_Tx_Ext_ApplyFcn(3);
      mask Callback ident: NsiCan_Tx_Ext_ApplyFcn(4);
      mask Callback ident_type: NsiCan_Tx_Ext_ApplyFcn(5);
      mask Callback dlc: NsiCan_Tx_Ext_ApplyFcn(6);
      mask Callback signals: NsiCan_Tx_Ext_ApplyFcn(7);
      mask Callback is_physical: NsiCan_Tx_Ext_ApplyFcn(7);
      mask Callback is_canfd: NsiCan_Tx_Ext_ApplyFcn(7);
      mask Callback is_crc: NsiCan_Tx_Ext_ApplyFcn(7);
      mask Display: image(imread('nsi.bmp'));text(0.5, 0.3, 'TX_VCU_HW_IO_CAN1', 'horizontalAlignment', 'center', 'verticalAlignment', 'base');plot([0.05 0.05 0.05 0.05 0.05 0.05 0.05 0.05 0.05 0.05]); port_label('input',1, 'Console_RTD'); port_label('input',2, 'Console_X'); port_label('input',3, 'Consle_Y'); port_label('input',4, 'Console_Z'); port_label('input',5, 'Coolant_Pump_Fan'); port_label('input',6, 'Coolant_AccyFan'); port_label('input',7, 'Buzzer'); port_label('input',8, 'LV_Battery_Voltage'); port_label('input',9, 'LV_Battery_SOC'); port_label('input',10, 'AccyFanFreq');
  CanTx8 : S-Function  FunctionName=NsiCan_Tx_Ext  Parameters=data_can,channel,msg_name,ident,ident_type,dlc,signals,is_physical,is_canfd,is_crc  SFunctionDeploymentMode=off  EnableBusSupport=off  mask(MUXlink Can Tx){data_can=1;HIGH_SPEED;500Kbps;No;C:\Users\TBRe-admin\Documents\Database\TBRe19_DBC_190620.dbc;0;;;0;HIGH_SPEED;500Kbps;120 Ohm;C:\Users\TBRe-admin\Documents\Database\TBRe19_DBC_190517.dbc;0;;;0;HIGH_SPEED;1000Kbps;120 Ohm;D:\TOOLS\MUXLINK\R2011b\MUXlink\misc\BASE_CAN_MUXLAB4.dbc;0;;;0;HIGH_SPEED;500Kbps;120 Ohm;D:\TOOLS\MUXLINK\R2011b\MUXlink\misc\j1939_adapt.dbc;0;;;0;HIGH_SPEED;1000Kbps;No;D:\TOOLS\MUXLINK\R2011b\MUXlink\misc\BASE_CAN_MUXLAB4.dbc;0;;, channel=1, msg_name=VCU_Vehicle_Functionality, ident=0x704, ident_type=STD, dlc=4, signals=Tractive_System_Startup;1;24;1;1.000000;0.000000;_;Throttle_Bool;1;25;1;1.000000;0.000000;_;MCU_NMT_Mode;1;16;8;1.000000;0.000000;_;Control_Word;1;0;8;1.000000;0.000000;_;Vehicle_Operation;1;8;8;1.000000;0.000000;_;Brake_Bool;1;26;1;1.000000;0.000000;_, is_physical=0, is_canfd=0, is_crc=0}
      mask prompts: data_can "data can"; msg_name "msg name"
      mask help: Transmit a frame on a CAN Channel.
      mask init:
      | NsiCan_Tx_Ext_InitializationFcn();
      settings: OpenFcn=NsiCan_Tx_Ext_OpenFcn();
      mask Help:
      | eval('block=get_param(gcb, ''RTWdata'');')
      | web([docroot '\toolbox\MUXlink\html\blocks/' block.MUXlink_BlockType '.html'])
      mask Callback data_can: NsiCan_Tx_Ext_ApplyFcn(1);
      mask Callback channel: NsiCan_Tx_Ext_ApplyFcn(2);
      mask Callback msg_name: NsiCan_Tx_Ext_ApplyFcn(3);
      mask Callback ident: NsiCan_Tx_Ext_ApplyFcn(4);
      mask Callback ident_type: NsiCan_Tx_Ext_ApplyFcn(5);
      mask Callback dlc: NsiCan_Tx_Ext_ApplyFcn(6);
      mask Callback signals: NsiCan_Tx_Ext_ApplyFcn(7);
      mask Callback is_physical: NsiCan_Tx_Ext_ApplyFcn(7);
      mask Callback is_canfd: NsiCan_Tx_Ext_ApplyFcn(7);
      mask Callback is_crc: NsiCan_Tx_Ext_ApplyFcn(7);
      mask Display: image(imread('nsi.bmp'));text(0.5, 0.3, 'TX_VCU_Vehicle_Functionality_CAN1', 'horizontalAlignment', 'center', 'verticalAlignment', 'base');plot([0.05 0.05 0.05 0.05 0.05 0.05 0.05 0.05 0.05 0.05]); port_label('input',1, 'Tractive_System_Startup'); port_label('input',2, 'Throttle_Bool'); port_label('input',3, 'MCU_NMT_Mode'); port_label('input',4, 'Control_Word'); port_label('input',5, 'Vehicle_Operation'); port_label('input',6, 'Brake_Bool');
  CanTx9 : S-Function  FunctionName=NsiCan_Tx_Ext  Parameters=data_can,channel,msg_name,ident,ident_type,dlc,signals,is_physical,is_canfd,is_crc  SFunctionDeploymentMode=off  EnableBusSupport=off  mask(MUXlink Can Tx){data_can=1;HIGH_SPEED;500Kbps;No;C:\Users\TBRe-admin\Documents\Database\TBRe19_DBC_190621.dbc;0;;;0;HIGH_SPEED;500Kbps;120 Ohm;C:\Users\TBRe-admin\Documents\Database\TBRe19_DBC_190517.dbc;0;;;0;HIGH_SPEED;1000Kbps;120 Ohm;D:\TOOLS\MUXLINK\R2011b\MUXlink\misc\BASE_CAN_MUXLAB4.dbc;0;;;0;HIGH_SPEED;500Kbps;120 Ohm;D:\TOOLS\MUXLINK\R2011b\MUXlink\misc\j1939_adapt.dbc;0;;;0;HIGH_SPEED;1000Kbps;No;D:\TOOLS\MUXLINK\R2011b\MUXlink\misc\BASE_CAN_MUXLAB4.dbc;0;;, channel=1, msg_name=VCU_Pedal_Voltages, ident=0x703, ident_type=STD, dlc=8, signals=Throttle1_Voltage;1;0;16;1.000000;0.000000;mV;Throttle2_Voltage;1;32;16;1.000000;0.000000;mV;Brake1_Voltage;1;16;16;1.000000;0.000000;mV;Brake2_Voltage;1;48;16;1.000000;0.000000;mV, is_physical=0, is_canfd=0, is_crc=0}
      mask prompts: data_can "data can"; msg_name "msg name"
      mask help: Transmit a frame on a CAN Channel.
      mask init:
      | NsiCan_Tx_Ext_InitializationFcn();
      settings: OpenFcn=NsiCan_Tx_Ext_OpenFcn();
      mask Help:
      | eval('block=get_param(gcb, ''RTWdata'');')
      | web([docroot '\toolbox\MUXlink\html\blocks/' block.MUXlink_BlockType '.html'])
      mask Callback data_can: NsiCan_Tx_Ext_ApplyFcn(1);
      mask Callback channel: NsiCan_Tx_Ext_ApplyFcn(2);
      mask Callback msg_name: NsiCan_Tx_Ext_ApplyFcn(3);
      mask Callback ident: NsiCan_Tx_Ext_ApplyFcn(4);
      mask Callback ident_type: NsiCan_Tx_Ext_ApplyFcn(5);
      mask Callback dlc: NsiCan_Tx_Ext_ApplyFcn(6);
      mask Callback signals: NsiCan_Tx_Ext_ApplyFcn(7);
      mask Callback is_physical: NsiCan_Tx_Ext_ApplyFcn(7);
      mask Callback is_canfd: NsiCan_Tx_Ext_ApplyFcn(7);
      mask Callback is_crc: NsiCan_Tx_Ext_ApplyFcn(7);
      mask Display: image(imread('nsi.bmp'));text(0.5, 0.3, 'TX_VCU_Pedal_Voltages_CAN1', 'horizontalAlignment', 'center', 'verticalAlignment', 'base');plot([0.05 0.05 0.05 0.05 0.05 0.05 0.05 0.05 0.05 0.05]); port_label('input',1, 'Throttle1_Voltage'); port_label('input',2, 'Throttle2_Voltage'); port_label('input',3, 'Brake1_Voltage'); port_label('input',4, 'Brake2_Voltage');
  Data Type Conversion{2..11,13..15,17,21..22,26..30,32} (22 alike) : DataTypeConversion
  Init : Subsystem  mask(System Initialize){}
      mask help: Add code to a systems Initialize function
      settings: CopyFcn=cccopyfcn(gcb)  OpenFcn=ccopenfcn('System Initialize Function')
      mask Help: This block contains text fields to insert custom user code sections at the declaration, execution and exit sections of the systems initialize function.  By placing this block inside a subsytem, the custom user code will appear in that subsystems function.
      mask Display: disp('I()')
  Task : S-Function  FunctionName=NsiSys_TaskREF  Parameters=task_initialised,task_periodic, task_sampletime,task_name,task_event,task_offset  SFunctionDeploymentMode=off  EnableBusSupport=off  mask(task definition){task_initialised=on, task_periodic=on, task_sampletime=[0.1], task_offset=0.01, task_name=DiagCAN4, task_event=on}
      mask prompts: task_initialised "task initialised"; task_periodic "Is Periodic"; task_sampletime "Task sample time"; task_offset "Task Offset"; task_name "Task name"; task_event "Is event"
      mask help:
      | Permit to provide all parameters associated to a MUXLINK task.
      | Task can be executed periodicaly and/or on event detection.
      | If task is periodic:
      | Task sample time specify the execution period in mS [0.001   6000]
      | Task Offset specify the offset applied to the execution period
      | Task Offset < Task sample time
      mask init:
      | NsiSys_TaskREF_InitializationFcn();
      settings: OpenFcn=NsiSys_Task_OpenFcn();
      mask Callback task_initialised: NsiSys_TaskREF_ApplyFcn(1);
      mask Callback task_periodic: NsiSys_TaskREF_ApplyFcn(2);
      mask Callback task_sampletime: NsiSys_TaskREF_ApplyFcn(3);
      mask Callback task_offset: NsiSys_TaskREF_ApplyFcn(6);
      mask Callback task_name: NsiSys_TaskREF_ApplyFcn(4);
      mask Callback task_event: NsiSys_TaskREF_ApplyFcn(5);
      mask Display: text(0.5, 0.8, 't()', 'horizontalAlignment', 'center', 'verticalAlignment', 'base');text(0.5, 0.2, '/ 100.0ms / 10.0ms /', 'horizontalAlignment', 'center', 'verticalAlignment', 'base');text(0.5, 0.4, 'Event', 'horizontalAlignment', 'center', 'verticalAlignment', 'base');
  UsbRx : S-Function  FunctionName=NsiUsb_Rx  Parameters=signame,sigtype,resolution,offset,unite,value,is_trigger  SFunctionDeploymentMode=off  EnableBusSupport=off  mask(MUXlink Usb Rx){signame=Wheel_Size, sigtype=Unsigned Byte, resolution=1, offset=0, unite=mm, value=450, is_trigger=off}
      mask prompts: signame "Signal name :"; sigtype "Signal type :"; resolution "Resolution :"; offset "Offset :"; unite "Unit :"; value "Default value :"; is_trigger "Is trigger ?"
      mask help: Receive a frame on the USB Channel.
      mask init:
      | NsiUsb_Rx_InitializationFcn();
      settings: OpenFcn=NsiUsb_Rx_OpenFcn();
      mask Help:
      | eval('block=get_param(gcb, ''RTWdata'');')
      | web([docroot '\toolbox\MUXlink\html\blocks/' block.MUXlink_BlockType '.html'])
      mask Callback signame: NsiUsb_Rx_ApplyFcn(1);
      mask TypeOptions sigtype: Boolean | Signed Byte | Unsigned Byte | Signed Word | Unsigned Word | Signed Double Word | Unsigned Double Word | Single Float | Double Float
      mask Callback sigtype: NsiUsb_Rx_ApplyFcn(2);
      mask Callback resolution: NsiUsb_Rx_ApplyFcn(3);
      mask Callback offset: NsiUsb_Rx_ApplyFcn(4);
      mask Callback unite: NsiUsb_Rx_ApplyFcn(5);
      mask Callback value: NsiUsb_Rx_ApplyFcn(6);
      mask Callback is_trigger: NsiUsb_Rx_ApplyFcn(7);
      mask Display: image(imread('nsi.bmp'));text(0.5, 0.2, 'USB Rx', 'horizontalAlignment', 'center', 'verticalAlignment', 'base');plot([0.05 0.05 0.05 0.05 0.05 0.05 0.05 0.05 0.05 0.05]);port_label('output',1, 'Wheel_Size');
  UsbRx1 : S-Function  FunctionName=NsiUsb_Rx  Parameters=signame,sigtype,resolution,offset,unite,value,is_trigger  SFunctionDeploymentMode=off  EnableBusSupport=off  mask(MUXlink Usb Rx){signame=Gearing_Ratio, sigtype=Unsigned Byte, resolution=1, offset=0, unite=ratio, value=3, is_trigger=off}
      mask prompts: signame "Signal name :"; sigtype "Signal type :"; resolution "Resolution :"; offset "Offset :"; unite "Unit :"; value "Default value :"; is_trigger "Is trigger ?"
      mask help: Receive a frame on the USB Channel.
      mask init:
      | NsiUsb_Rx_InitializationFcn();
      settings: OpenFcn=NsiUsb_Rx_OpenFcn();
      mask Help:
      | eval('block=get_param(gcb, ''RTWdata'');')
      | web([docroot '\toolbox\MUXlink\html\blocks/' block.MUXlink_BlockType '.html'])
      mask Callback signame: NsiUsb_Rx_ApplyFcn(1);
      mask TypeOptions sigtype: Boolean | Signed Byte | Unsigned Byte | Signed Word | Unsigned Word | Signed Double Word | Unsigned Double Word | Single Float | Double Float
      mask Callback sigtype: NsiUsb_Rx_ApplyFcn(2);
      mask Callback resolution: NsiUsb_Rx_ApplyFcn(3);
      mask Callback offset: NsiUsb_Rx_ApplyFcn(4);
      mask Callback unite: NsiUsb_Rx_ApplyFcn(5);
      mask Callback value: NsiUsb_Rx_ApplyFcn(6);
      mask Callback is_trigger: NsiUsb_Rx_ApplyFcn(7);
      mask Display: image(imread('nsi.bmp'));text(0.5, 0.2, 'USB Rx', 'horizontalAlignment', 'center', 'verticalAlignment', 'base');plot([0.05 0.05 0.05 0.05 0.05 0.05 0.05 0.05 0.05 0.05]);port_label('output',1, 'Gearing_Ratio');
  wires:
  Data Type Conversion7/1 -> CanTx6/2
  UsbRx/1 -> CanTx2/11
  Bus Selector/1 -> Data Type Conversion4/1  "<Throttle1_Voltage>"
  Bus Selector/3 -> Data Type Conversion3/1  "<Brake1_Pressure>"
  Data Type Conversion14/1 -> CanTx6/1
  Data Type Conversion3/1 -> CanTx9/3
  Bus Selector4/1 -> Data Type Conversion27/1  "<AIRLow>"
  Data Type Conversion26/1 -> CanTx2/3
  Bus Selector2/2 -> CanTx7/2  "<btnX_Input>"
  Bus Selector2/6 -> CanTx7/6  "<AccyFanPower>"
  Bus Selector2/5 -> CanTx7/5  "<PumpFanPower>"
  Data Type Conversion27/1 -> CanTx2/2
  Bus Selector4/6 -> Data Type Conversion30/1  "<APPS_BP_Implausibility>"
  Data Type Conversion28/1 -> CanTx2/4
  Bus Selector4/2 -> Data Type Conversion26/1  "<AIRHigh>"
  Data Type Conversion13/1 -> CanTx7/8
  Data Type Conversion5/1 -> CanTx6/7
  Bus Selector4/5 -> Data Type Conversion29/1  "<APPS_Implausibility>"
  Bus Selector2/4 -> CanTx7/4  "<btnZ_Input>"
  Bus Selector1/2 -> Data Type Conversion7/1  "<Brake2_Per>"
  Data Type Conversion2/1 -> CanTx9/2
  Data Type Conversion10/1 -> CanTx6/5
  Data Type Conversion21/1 -> CanTx8/6
  Bus Selector4/7 -> Data Type Conversion32/1  "<LV_Warning>"
  Bus Selector4/4 -> Data Type Conversion11/1  "<Pedal_Sensor_Fail>"
  Bus Selector1/6 -> Data Type Conversion5/1  "<Throttle_Percentage>"
  Bus Selector1/4 -> Data Type Conversion10/1  "<Throttle1_Per>"
  Data Type Conversion17/1 -> CanTx8/2
  PostPL_Bus/1 -> Bus Selector/1, Bus Selector1/1, Bus Selector2/1, Bus Selector4/1, Bus Selector3/1
  Data Type Conversion8/1 -> CanTx6/3
  Data Type Conversion9/1 -> CanTx6/6
  Data Type Conversion29/1 -> CanTx2/6
  Data Type Conversion6/1 -> CanTx9/4
  Bus Selector2/1 -> CanTx7/1  "<btnRTD_Input>"
  Bus Selector/2 -> Data Type Conversion2/1  "<Throttle2_Voltage>"
  Data Type Conversion15/1 -> CanTx7/9
  Data Type Conversion30/1 -> CanTx2/7
  Bus Selector2/3 -> CanTx7/3  "<btnY_Input>"
  Data Type Conversion4/1 -> CanTx9/1
  Bus Selector4/3 -> Data Type Conversion28/1  "<BPPS_Implausibility>"
  Bus Selector3/1 -> Data Type Conversion17/1  "<Throttle_Bool>"
  Bus Selector2/8 -> Data Type Conversion15/1  "<LV_SOC%>"
  Bus Selector2/9 -> Data Type Conversion22/1  "<Fan_Freq>"
  UsbRx1/1 -> CanTx2/10
  Data Type Conversion11/1 -> CanTx2/5
  Bus Selector3/2 -> Data Type Conversion21/1  "<Brake_Bool>"
  Data Type Conversion32/1 -> CanTx2/9
  Bus Selector2/7 -> Data Type Conversion13/1  "<LV_Battery_Voltage>"
  Bus Selector1/5 -> Data Type Conversion9/1  "<Throttle2_Per>"
  Bus Selector1/3 -> Data Type Conversion8/1  "<Brake_Percentage>"
  Data Type Conversion22/1 -> CanTx7/10
  Bus Selector1/1 -> Data Type Conversion14/1  "<Brake1_Per>"
  Bus Selector/4 -> Data Type Conversion6/1  "<Brake2_Pressure>"
